simulink model "BatteryHV_testHarness"  (R2020b)
settings: Solver=VariableStepAuto  StartTime=0.0  StopTime=500  RelTol=1e-3  AbsTol=1e-3
PreLoadFcn:
  | BatteryHV_testParams
libraries: fl_lib x2, nesl_utility x2
settings Model: EnablePacing=on  PacingRate=6  Creator=isaacito  LastModifiedBy=isaacito
settings SolverCC: AutoScaleAbsTol=off
settings SimscapeCC: SimscapeLogType=local  SimscapeLogSimulationStatistics=on  SimscapeLogToSDI=on  SimscapeLogLimitData=off

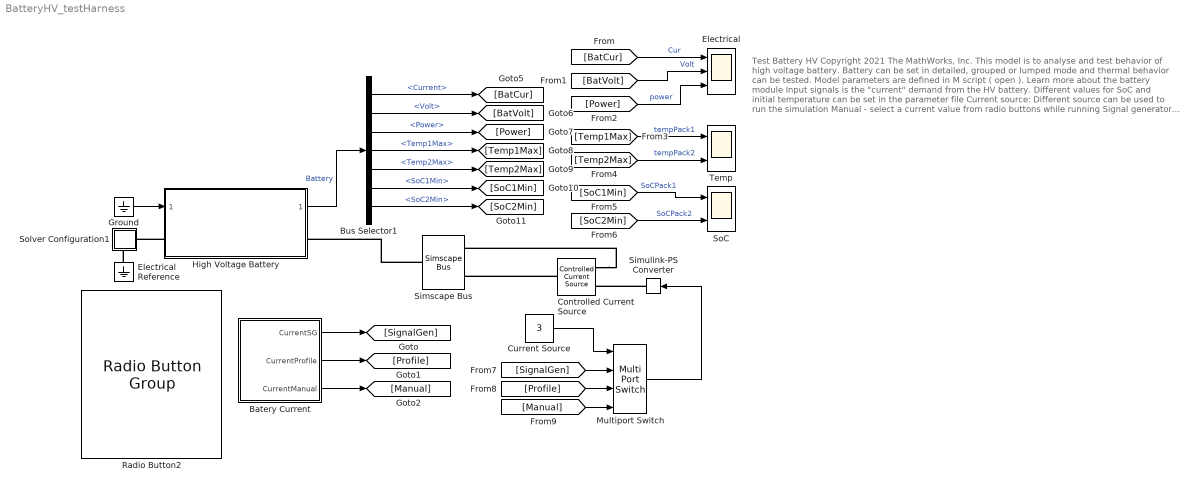
== system BatteryHV_testHarness ==
  note: Test Battery HV
      |
      | Copyright 2021 The MathWorks, Inc.
      |
      | This model is to analyse and test behavior of high voltage battery. Battery can be set in detailed, grouped or lumped mode and thermal behavior can be tested.
      |
      | Model parameters are defined in M script ( open ).
      | Learn more about the battery module
      |
      | Input signals is the "current" demand from the HV battery.
      | Different values for SoC and initial temperature can be set in the parameter file
      |
      | Current source: Different source can be used to run the simulation
      | Manual - select a current value from radio buttons while running
      | Signal generator - standard waveforms can be selected
      | Profile - current data from some standard drive runs are used
      |
      | Note that Simulation Pacing is enabled for simulation. While
      | simulation is running, select current in radio button, and observe the SoC Min, Temp Max and battery voltage.
      | Input and output signal are also logged during simulation.
      | Use Data Inspector to plot the logged signals.
  " Simscape Bus" : SimscapeBus  HierarchyStrings=plus;minus
  Batery Current : Subsystem
  Bus Selector1 : BusSelector  OutputSignals=Current,Volt,Power,Temp1Max,Temp2Max,SoC1Min,SoC2Min
  Controlled Current Source : fl_lib/Electrical/Electrical Sources/Controlled Current Source
  Current Source : Constant  Value=3
  Electrical : Scope  NumInputPorts=3
  Electrical Reference : fl_lib/Electrical/Electrical Elements/Electrical Reference
  Ground : Ground
  High Voltage Battery : Subsystem  ReferencedSubsystem=BatteryHVPackRefSub
  Multiport Switch : MultiPortSwitch
  Radio Button2 : RadioButtonGroup  LabelPosition=Bottom  SelectedLabel=50 A  ButtonGroupName=Group
      settings: Values={{'-100 A', '-50 A', '-10 A', '0 A', '10 A', '50 A', '100 A'}, [-100 -50 -10 0 10 50 100]}
  Simulink-PS Converter : nesl_utility/Simulink-PS Converter  PhysicalDomain=network_engine_domain  SubClassName=ps_input  LeftPortType=input  RightPortType=output  PseudoPeriodic=off  Frequencies=[]  NoiseDistribution=none  NoiseParameters=[]  Unit=1  AffineConversion=off  FilteringAndDerivatives=provide  SimscapeFilterOrder=1  InputFilterTimeConstant=0.001  UdotUserProvided=0
  SoC : Scope  NumInputPorts=2
  Solver Configuration1 : Subsystem
      settings: PortSchema="{\"entries\":[{\"content\":{\"sides\":[{\"content\":{\"connectorIds\":[]},\"type\":\"ConnectorPlacement.EquallySpacedRectSide\",\"uuid\":\"4a7e26c2-e9e9-4fea-b605-533b1a682be7\"},{\"content\":{\"connectorIds\":[\"RConn1\"],\"side\":\"RIGHT\"},\"type\":\"ConnectorPlacement.EquallySpacedRectSide\",\"uuid\":\"0210e324-555e-4372-b836-fcc8ab23e933\"},{\"content\":{\"connectorIds\":[],\"side\":\"TOP\"},\"type\":\"ConnectorPlacement.EquallySpacedRectSide\",\"uuid\":\"9bbae011-e6fc-4534-a44f-d79a5697c939\"},{\"content\":{\"connectorIds\":[\"RConn2\"],\"side\":\"BOTTOM\"},\"type\":\"ConnectorPlacement.EquallySpacedRectSide\",\"uuid\":\"d5829c0a-26ea-402d-a1c6-900997ddf1a8\"}]},\"type\":\"ConnectorPlacement.EquallySpacedConnector\",\"uuid\":\"f4e17c65-54c6-42fe-a467-9c6b014b697a\"}],\"packageUris\":[\"http://schema.mathworks.com/mf0/Connector/19700101\"],\"version\":\"1.0\"}"
  Temp : Scope  NumInputPorts=2
  wires:
  High Voltage Battery/1 -> Bus Selector1/1  "Battery"
  Ground/1 -> High Voltage Battery/1
  Bus Selector1/1 -> [BatCur]  "<Current>"
  Bus Selector1/2 -> [BatVolt]  "<Volt>"
  Bus Selector1/3 -> [Power]  "<Power>"
  Bus Selector1/4 -> [Temp1Max]  "<Temp1Max>"
  Bus Selector1/5 -> [Temp2Max]  "<Temp2Max>"
  Bus Selector1/6 -> [SoC1Min]  "<SoC1Min>"
  Bus Selector1/7 -> [SoC2Min]  "<SoC2Min>"
  [BatVolt] -> Electrical/2  "Volt"
  [BatCur] -> Electrical/1  "Cur"
  [Power] -> Electrical/3  "power"
  [Temp1Max] -> Temp/1  "tempPack1"
  [Temp2Max] -> Temp/2  "tempPack2"
  [SoC1Min] -> SoC/1  "SoCPack1"
  [SoC2Min] -> SoC/2  "SoCPack2"
  Batery Current/1(CurrentSG) -> [SignalGen]
  Batery Current/3(CurrentManual) -> [Manual]
  Batery Current/2(CurrentProfile) -> [Profile]
  [SignalGen] -> Multiport Switch/2
  [Profile] -> Multiport Switch/3
  [Manual] -> Multiport Switch/4
  Multiport Switch/1 -> Simulink-PS Converter/1
  Current Source/1 -> Multiport Switch/1
  connections:
  Electrical Reference/LConn1 -- Solver Configuration1/RConn2
  High Voltage Battery/LConn1 -- Solver Configuration1/RConn1
  " Simscape Bus"/RConn1 -- High Voltage Battery/RConn1
  Controlled Current Source/RConn2 -- " Simscape Bus"/LConn1
  Simulink-PS Converter/RConn1 -- Controlled Current Source/RConn1
  Controlled Current Source/LConn1 -- " Simscape Bus"/LConn2

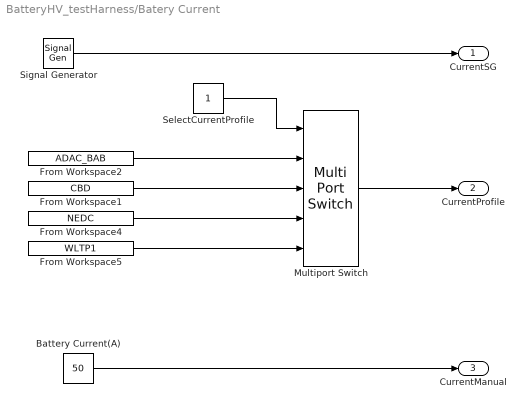
== system BatteryHV_testHarness/Batery Current ==
  Battery Current(A) : Constant  Value=50
  From Workspace1 : FromWorkspace  VariableName=CBD
  From Workspace2 : FromWorkspace  VariableName=ADAC_BAB
  From Workspace4 : FromWorkspace  VariableName=NEDC
  From Workspace5 : FromWorkspace  VariableName=WLTP1
  Multiport Switch : MultiPortSwitch  Inputs=4
  SelectCurrentProfile : Constant
  Signal Generator : SignalGenerator  WaveForm=square  Amplitude=20  Frequency=0.05  Units=rad/sec
  CurrentSG : Outport
  CurrentProfile : Outport  Port=2
  CurrentManual : Outport  Port=3
  wires:
  Signal Generator/1 -> CurrentSG/1
  From Workspace2/1 -> Multiport Switch/2
  From Workspace1/1 -> Multiport Switch/3
  From Workspace4/1 -> Multiport Switch/4
  Multiport Switch/1 -> CurrentProfile/1
  SelectCurrentProfile/1 -> Multiport Switch/1
  From Workspace5/1 -> Multiport Switch/5
  Battery Current(A)/1 -> CurrentManual/1

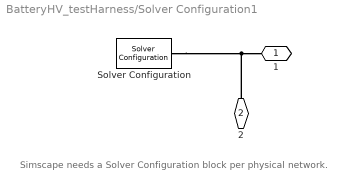
== system BatteryHV_testHarness/Solver Configuration1 ==
  note: Simscape needs a Solver Configuration block per physical network.
  Solver Configuration : nesl_utility/Solver Configuration  PhysicalDomain=network_engine_domain  SubClassName=solver  LeftPortType=input  RightPortType=generic  Tones=[]  Harmonics=[]  SimulateNoise=off  Profile=off  UseLocalSampling=off  EnableSwitchedLinearOptims=on  FrequencyDomain=off  UseCCode=off  RelTol=0.001  AbsTol=1e-06  MinStep=1e-09  ToWorkspace=off  RevertToSquareIcSolve=off  NumHomotopyIterations=100  PhasorMode=off  PhasorModeNumHarmonics=1  DoDC=off  ResidualTolerance=1e-9  UseLocalSolver=off  LocalSolverChoice=NE_BACKWARD_EULER_ADVANCER  LocalSolverSampleTime=0.01  DoFixedCost=off  MaxNonlinIter=3  MaxModeIter=2  ComputeImpulses=off  ImpulseIterations=2  LinearAlgebra=auto  EquationFormulation=NE_TIME_EF  DelaysMemoryBudget=1024  AutomaticFiltering=on  FilteringTimeConstant=0.001  PartitionStorageMethod=AS_NEEDED  PartitionMemoryBudget=1024  PartitionMethod=FAST
      settings: AttributesFormatString=Local solver %<UseLocalSolver>
  1 : PMIOPort  Side=Right
  2 : PMIOPort  Port=2  Side=Right
  connections:
  Solver Configuration/RConn1 -- 1/RConn1 -- 2/RConn1
